simulink model "ball_and_beam_c"  (R2016a)
settings: Solver=VariableStepAuto  StartTime=0.0  StopTime=10.0  RelTol=1e-3
undefined symbols (not defined in the file): dq0, g, Ja, L, M, m, q0
settings Model: Creator=mgreiff  LastModifiedBy=mgreiff
settings DataIOCC: LimitDataPoints=on
settings DebuggingCC: AllowSymbolicDim=off
settings ModelReferenceCC: PropagateSignalLabelsOutOfModel=off
settings GRTTargetCC: GeneratePreprocessorConditionals=Use local settings

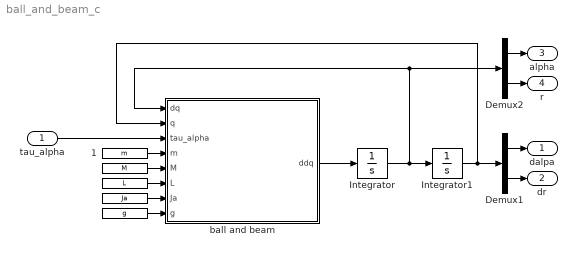
== system ball_and_beam_c ==
  tau_alpha : Inport  PortDimensions=1
  " " : Constant  Value=L
  "  " : Constant  Value=Ja
  "   " : Constant  Value=g
  "        " : Constant  Value=M
  " 1" : Constant  Value=m
  Demux1 : Demux  Outputs=2
  Demux2 : Demux  Outputs=2
  Integrator : Integrator  InitialCondition=dq0
  Integrator1 : Integrator  InitialCondition=q0
  ball and beam : MATLAB Function  TreatAsAtomicUnit=on
  "dalpa " : Outport  PortDimensions=1
  dr : Outport  Port=2  PortDimensions=1
  alpha : Outport  Port=3  PortDimensions=1
  r : Outport  Port=4  PortDimensions=1
  wires:
  ball and beam/1(ddq) -> Integrator/1
  Integrator/1 -> Demux2/1, ball and beam/1(dq), Integrator1/1
  Integrator1/1 -> ball and beam/2(q), Demux1/1
  tau_alpha/1 -> ball and beam/3(tau_alpha)
  " "/1 -> ball and beam/6(L)
  "  "/1 -> ball and beam/7(Ja)
  "   "/1 -> ball and beam/8(g)
  Demux1/2 -> dr/1
  Demux1/1 -> "dalpa "/1
  Demux2/2 -> r/1
  Demux2/1 -> alpha/1
  " 1"/1 -> ball and beam/4(m)
  "        "/1 -> ball and beam/5(M)

== matlab function ball_and_beam_c/ball and beam ==
  data: dq input; q input; tau_alpha input; m input; M input; ddq output; L input; Ja input; g input
function ddq = fcn(dq, q, tau_alpha, m, M, L, Ja, g)
%#codegen
alpha  = q(1);
r      = q(2);
dalpha = dq(1);
dr     = dq(2);

ddalpha = (tau_alpha...
           -2 * m * r * dr * dalpha + ...
           -(m * g * r + L * M *g) * cos(alpha))/...
           (Ja + m*r^2);
ddr = (5/7) * (r*dalpha - g * sin(alpha));
ddq = [ddalpha; ddr];
end
